simulink model "xxx"  (R2016a)
settings: Solver=VariableStepAuto  StartTime=0.0  StopTime=10.0  RelTol=1e-3
undefined symbols (not defined in the file): A, a1, a2, A3, A4, b1, b2, beta, c1, c2, Cppx, Cppy, Cpx, Cpy, M, m, R1, R2, R4, RL, V4, V5, VA, VB
settings Model: Creator=xlh  LastModifiedBy=xlh

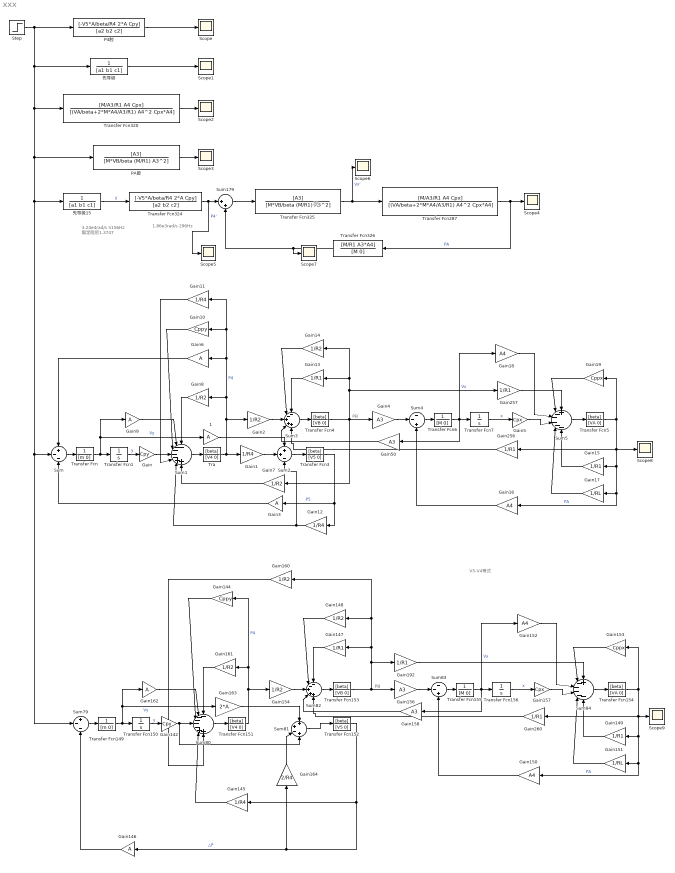
== system xxx ==
  note: 1.86e3rad/s
      | 296Hz
  note: PB
  note: 3.24e4rad/s
      | 5156Hz
      | 固定阻尼1.3747
  note: PB
  note: V5-V4等式
  note: PB
  1 : Gain  Gain=A
  Gain : Gain  Gain=Cpy
  Gain{1,11..12,145} (4 alike) : Gain  Gain=1/R4
  Gain10 : Gain  Gain=Cppy
  Gain{13,15,147,149,192,256..257,260} (8 alike) : Gain  Gain=1/R1
  Gain{2,7..8,14,148,154,160..161} (8 alike) : Gain  Gain=1/R2
  Gain142 : Gain  Gain=Cpy
  Gain144 : Gain  Gain=Cppy
  Gain{3,6,9,146,162} (5 alike) : Gain  Gain=A
  Gain{16,18,150,152} (4 alike) : Gain  Gain=A4
  Gain151 : Gain  Gain=1/RL
  Gain153 : Gain  Gain=Cppx
  Gain{4,50,156,158} (4 alike) : Gain  Gain=A3
  Gain157 : Gain  Gain=Cpx
  Gain163 : Gain  Gain=2*A
  Gain164 : Gain  Gain=2/R4
  Gain17 : Gain  Gain=1/RL
  Gain19 : Gain  Gain=Cppx
  Gain5 : Gain  Gain=Cpx
  P4腔 : TransferFcn  Numerator=[-V5*A/beta/R4 2*A Cpy]  Denominator=[a2 b2 c2]
  PA腔 : TransferFcn  Numerator=[A3]  Denominator=[M*VB/beta (M/R1) A3^2]
  Scope{,1..9} (10 alike) : Scope
  Step : Step  SampleTime=0
  Sum : Sum  Inputs=+--
  Sum1 : Sum  Inputs=-----++
  Sum179 : Sum  Inputs=|++
  Sum2 : Sum  Inputs=++-
  Sum3 : Sum  Inputs=--+++
  Sum4 : Sum  Inputs=--+
  Sum5 : Sum  Inputs=+-----
  Sum79 : Sum  Inputs=+--
  Sum80 : Sum  Inputs=-----++
  Sum81 : Sum  Inputs=++-+
  Sum82 : Sum  Inputs=--+++
  Sum83 : Sum  Inputs=--+
  Sum84 : Sum  Inputs=+-----
  Tra : TransferFcn  Numerator=[beta]  Denominator=[V4 0]
  Transfer Fcn : TransferFcn  Denominator=[m 0]
  Transfer Fcn{1,7,150,156} (4 alike) : TransferFcn  Denominator=[1 0]
  Transfer Fcn149 : TransferFcn  Denominator=[m 0]
  Transfer Fcn151 : TransferFcn  Numerator=[beta]  Denominator=[V4 0]
  Transfer Fcn152 : TransferFcn  Numerator=[beta]  Denominator=[V5 0]
  Transfer Fcn153 : TransferFcn  Numerator=[beta]  Denominator=[VB 0]
  Transfer Fcn154 : TransferFcn  Numerator=[beta]  Denominator=[VA 0]
  Transfer Fcn155 : TransferFcn  Denominator=[M 0]
  Transfer Fcn287 : TransferFcn  Numerator=[M/A3/R1 A4 Cpx]  Denominator=[(VA/beta+2*M*A4/A3/R1) A4^2 Cpx*A4]
  Transfer Fcn3 : TransferFcn  Numerator=[beta]  Denominator=[V5 0]
  Transfer Fcn320 : TransferFcn  Numerator=[M/A3/R1 A4 Cpx]  Denominator=[(VA/beta+2*M*A4/A3/R1) A4^2 Cpx*A4]
  Transfer Fcn324 : TransferFcn  Numerator=[-V5*A/beta/R4 2*A Cpy]  Denominator=[a2 b2 c2]
  Transfer Fcn325 : TransferFcn  Numerator=[A3]  Denominator=[M*VB/beta (M/R1) A3^2]
  Transfer Fcn326 : TransferFcn  Numerator=[M/R1 A3*A4]  Denominator=[M 0]
  Transfer Fcn4 : TransferFcn  Numerator=[beta]  Denominator=[VB 0]
  Transfer Fcn5 : TransferFcn  Numerator=[beta]  Denominator=[VA 0]
  Transfer Fcn6 : TransferFcn  Denominator=[M 0]
  先导级 : TransferFcn  Denominator=[a1 b1 c1]
  先导级15 : TransferFcn  Denominator=[a1 b1 c1]
  wires:
  P4腔/1 -> Scope/1
  先导级/1 -> Scope1/1
  Transfer Fcn320/1 -> Scope2/1
  PA腔/1 -> Scope3/1
  Sum179/1 -> Transfer Fcn325/1
  Transfer Fcn325/1 -> Scope6/1, Transfer Fcn287/1  "Vx'"
  Transfer Fcn287/1 -> Scope4/1, Transfer Fcn326/1  "PA"
  先导级15/1 -> Transfer Fcn324/1  "y"
  Transfer Fcn324/1 -> Scope5/1, Sum179/1  "P4'"
  Transfer Fcn326/1 -> Scope7/1, Sum179/2
  Sum/1 -> Transfer Fcn/1
  Transfer Fcn/1 -> Gain9/1, 1/1, Transfer Fcn1/1  "Vy"
  Transfer Fcn1/1 -> Gain/1  "y"
  Gain/1 -> Sum1/4
  Sum1/1 -> Tra/1
  Tra/1 -> Gain11/1, Gain10/1, Gain6/1, Gain8/1, Gain2/1, Gain1/1  "P4"
  Gain1/1 -> Sum2/2
  Sum2/1 -> Transfer Fcn3/1
  Transfer Fcn3/1 -> Gain12/1, Gain3/1  "P5"
  Gain3/1 -> Sum/3
  Gain2/1 -> Sum3/3
  Sum3/1 -> Transfer Fcn4/1
  Transfer Fcn4/1 -> Gain257/1, Gain14/1, Gain13/1, Gain7/1, Gain4/1
  Gain4/1 -> Sum4/2
  Sum4/1 -> Transfer Fcn6/1
  Transfer Fcn6/1 -> Gain50/1, Gain18/1, Transfer Fcn7/1  "Vx"
  Transfer Fcn7/1 -> Gain5/1  "x"
  Gain5/1 -> Sum5/4
  Sum5/1 -> Transfer Fcn5/1
  Transfer Fcn5/1 -> Gain256/1, Scope8/1, Gain16/1, Gain17/1, Gain15/1, Gain19/1  "PA"
  Gain6/1 -> Sum/1
  Gain7/1 -> Sum1/7
  Gain8/1 -> Sum1/1
  Gain9/1 -> Sum1/2
  Gain10/1 -> Sum1/3
  Gain11/1 -> Sum1/5
  Gain12/1 -> Sum1/6, Sum2/3
  Gain13/1 -> Sum3/1
  Gain14/1 -> Sum3/2
  Gain15/1 -> Sum5/6
  Gain16/1 -> Sum4/3
  Gain17/1 -> Sum5/5
  Gain18/1 -> Sum5/3
  Gain19/1 -> Sum5/2
  Gain50/1 -> Sum3/4
  Gain256/1 -> Sum3/5
  Gain257/1 -> Sum5/1
  1/1 -> Sum2/1
  Sum79/1 -> Transfer Fcn149/1
  Transfer Fcn149/1 -> Transfer Fcn150/1, Gain163/1, Gain162/1  "Vy"
  Gain142/1 -> Sum81/4, Sum80/4
  Step/1 -> P4腔/1, 先导级/1, Sum79/2, Sum/2, 先导级15/1, PA腔/1, Transfer Fcn320/1
  Sum80/1 -> Transfer Fcn151/1
  Transfer Fcn151/1 -> Gain154/1, Gain161/1, Gain144/1  "P4"
  Sum81/1 -> Transfer Fcn152/1
  Transfer Fcn152/1 -> Gain145/1, Gain146/1, Gain164/1  "△P"
  Gain154/1 -> Sum82/3
  Sum82/1 -> Transfer Fcn153/1
  Transfer Fcn153/1 -> Gain192/1, Gain160/1, Gain148/1, Gain147/1, Gain156/1
  Gain156/1 -> Sum83/2
  Sum83/1 -> Transfer Fcn155/1
  Transfer Fcn155/1 -> Transfer Fcn156/1, Gain152/1, Gain158/1  "Vx"
  Transfer Fcn156/1 -> Gain157/1  "x"
  Gain157/1 -> Sum84/4
  Sum84/1 -> Transfer Fcn154/1
  Transfer Fcn154/1 -> Gain153/1, Scope9/1, Gain260/1, Gain149/1, Gain151/1, Gain150/1  "PA"
  Gain160/1 -> Sum80/7
  Gain161/1 -> Sum80/1
  Gain162/1 -> Sum80/2
  Gain144/1 -> Sum80/3
  Gain147/1 -> Sum82/1
  Gain148/1 -> Sum82/2
  Gain149/1 -> Sum84/6
  Gain150/1 -> Sum83/3
  Gain151/1 -> Sum84/5
  Gain152/1 -> Sum84/3
  Gain153/1 -> Sum84/2
  Gain158/1 -> Sum82/4
  Gain163/1 -> Sum81/1
  Gain164/1 -> Sum81/3
  Transfer Fcn150/1 -> Gain142/1  "y"
  Gain145/1 -> Sum80/6
  Gain146/1 -> Sum79/3
  Gain192/1 -> Sum84/1
  Gain260/1 -> Sum82/5
